simulink model "MPC_no_v_w"  (R2020b)
settings: Solver=VariableStepAuto  StartTime=0.0  StopTime=400.0  RelTol=1e-3
values from neighbouring files (symbols this model uses):
  condtheta = x0(3)    [MPCprova_no_v_walker.m]
  condx = x0(1)    [MPCprova_no_v_walker.m]
  condy = x0(2)    [MPCprova_no_v_walker.m]
  x_ref = [0 0 0 0 0]    [MPCprova_no_v_walker.m]
libraries: mpclib x1
settings Model: Creator=adelina  LastModifiedBy=adelina

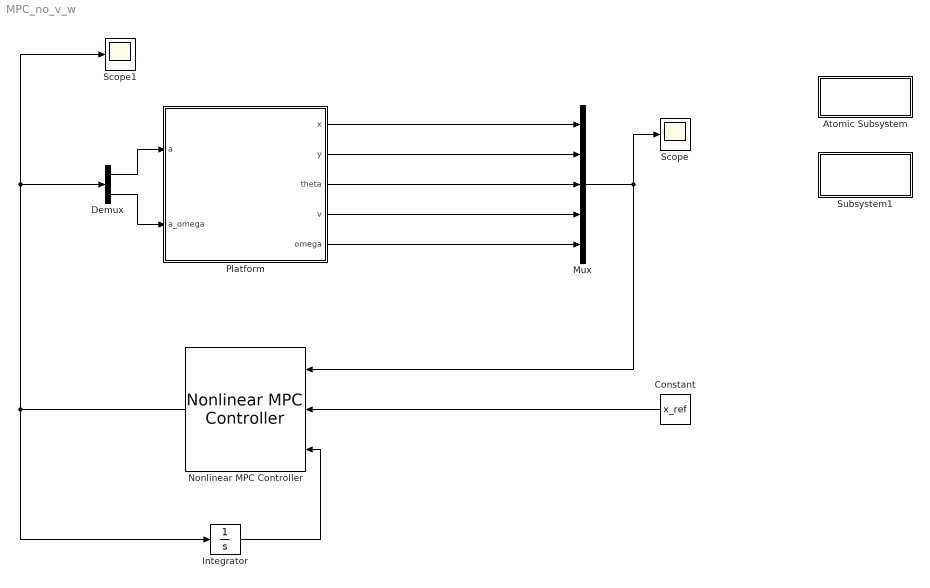
== system MPC_no_v_w ==
  Atomic Subsystem : Subsystem  TreatAsAtomicUnit=on
      settings: OpenFcn=MPCprova_no_v_walker
      mask Display: disp('initialization')
  Constant : Constant  Value=x_ref  VectorParams1D=off
  Demux : Demux  Outputs=2
  Integrator : Integrator
  Mux : Mux  Inputs=5
  Nonlinear MPC Controller : mpclib/Nonlinear MPC Controller  SCDEnableBlockLinearizationSpecification=on  nlmpcobj=nlobj  UseObjectTs=on  UseMEX=off  md_enabled=off  mvtarget_enabled=off  param_enabled=off  cost_enabled=off  mvseq_enabled=off  stateseq_enabled=off  ovseq_enabled=off  slack_enabled=off  status_enabled=off  ov_min=off  ov_max=off  mv_min=off  mv_max=off  mvrate_min=off  mvrate_max=off  state_min=off  state_max=off  ov_weight=off  mv_weight=off  mvrate_weight=off  ecr_weight=off  nlp_initialize=off
  Platform : Subsystem
  Scope : Scope
  Scope1 : Scope
  Subsystem1 : Subsystem
      settings: OpenFcn=plots
      mask Display: disp('plots')
  wires:
  Platform/1(x) -> Mux/1
  Platform/2(y) -> Mux/2
  Mux/1 -> Nonlinear MPC Controller/1, Scope/1
  Platform/3(theta) -> Mux/3
  Platform/4(v) -> Mux/4
  Platform/5(omega) -> Mux/5
  Nonlinear MPC Controller/1 -> Integrator/1, Scope1/1, Demux/1
  Demux/2 -> Platform/2(a_omega)
  Demux/1 -> Platform/1(a)
  Integrator/1 -> Nonlinear MPC Controller/3
  Constant/1 -> Nonlinear MPC Controller/2

== system MPC_no_v_w/Atomic Subsystem ==

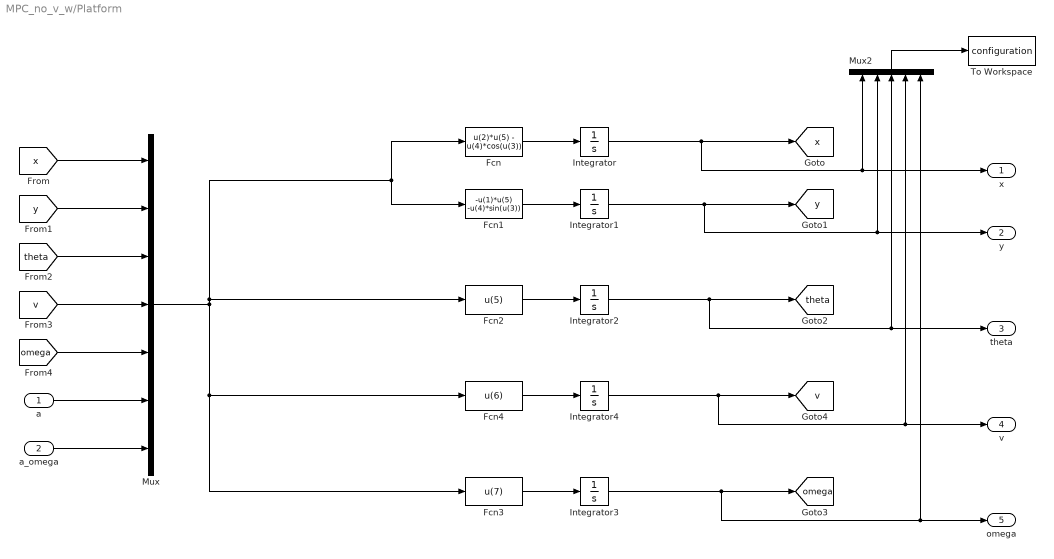
== system MPC_no_v_w/Platform ==
  a : Inport
  a_omega : Inport  Port=2
  Fcn : Fcn  Expr=u(2)*u(5) - u(4)*cos(u(3))
  Fcn1 : Fcn  Expr=-u(1)*u(5) -u(4)*sin(u(3))
  Fcn2 : Fcn  Expr=u(5)
  Fcn3 : Fcn  Expr=u(7)
  Fcn4 : Fcn  Expr=u(6)
  Integrator : Integrator  InitialCondition=condx
  Integrator1 : Integrator  InitialCondition=condy
  Integrator2 : Integrator  InitialCondition=condtheta
  Integrator3 : Integrator
  Integrator4 : Integrator
  Mux : Mux  Inputs=7
  Mux2 : Mux  Inputs=5
  To Workspace : ToWorkspace  VariableName=configuration  SaveFormat=Structure With Time  SampleTime=-1
  x : Outport
  y : Outport  Port=2
  theta : Outport  Port=3
  v : Outport  Port=4
  omega : Outport  Port=5
  tag scope: omega=global, theta=global, v=global, x=global, y=global
  wires:
  Fcn2/1 -> Integrator2/1
  Integrator2/1 -> [theta], theta/1, Mux2/3
  Fcn1/1 -> Integrator1/1
  [y] -> Mux/2
  [x] -> Mux/1
  a/1 -> Mux/6
  Integrator1/1 -> [y], y/1, Mux2/2
  [theta] -> Mux/3
  Integrator/1 -> x/1, Mux2/1, [x]
  Fcn/1 -> Integrator/1
  a_omega/1 -> Mux/7
  Mux2/1 -> To Workspace/1
  [v] -> Mux/4
  [omega] -> Mux/5
  Mux/1 -> Fcn3/1, Fcn4/1, Fcn1/1, Fcn/1, Fcn2/1
  Integrator3/1 -> [omega], omega/1, Mux2/5
  Fcn3/1 -> Integrator3/1
  Integrator4/1 -> v/1, Mux2/4, [v]
  Fcn4/1 -> Integrator4/1

== system MPC_no_v_w/Subsystem1 ==
